simulink model "tb_adc_5g_spi_sys"  (Simulink 7.0)
settings: Solver=ode45  StartTime=0.0  StopTime=2000  RelTol=1e-3
libraries: xbsIndex_r4 x446, simulink x28, xps_library x12, dspsigops x12, xbsReplacements_r4 x4, casper_library x2
(part 2 of 5)

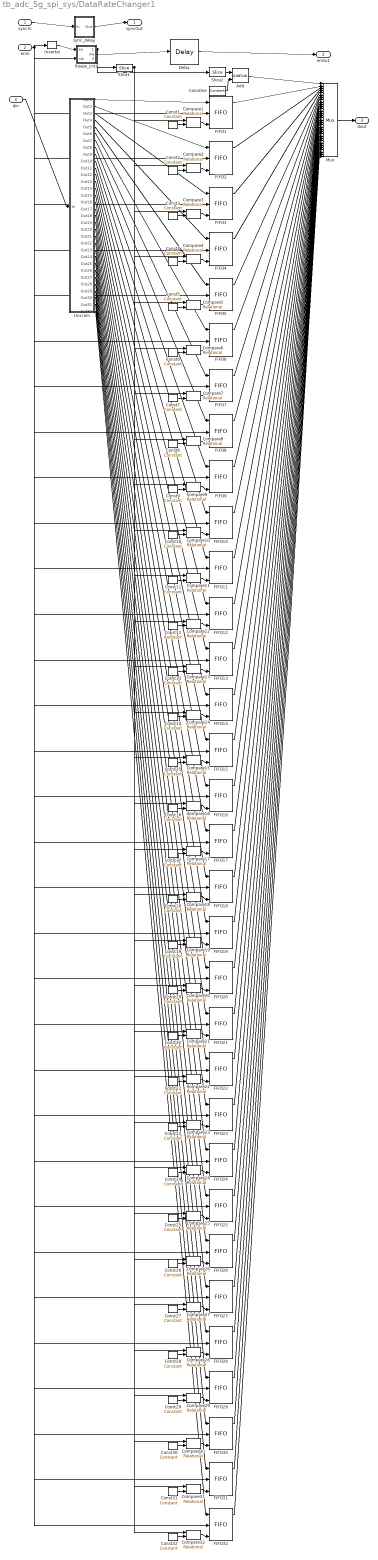
== system tb_adc_5g_spi_sys/DataRateChanger1 ==
  syncIn : Inport  OutDataType=sfix(16)  OutScaling=2^0
  enIn : Inport  Port=2  OutDataType=sfix(16)  OutScaling=2^0
  din : Inport  Port=3  OutDataType=sfix(16)  OutScaling=2^0
  Add : xbsIndex_r4/AddSub  mode=Addition  use_carryin=off  use_carryout=off  en=off  latency=0  precision=User Defined  arith_type=Unsigned  n_bits=5  bin_pt=0  quantization=Truncate  overflow=Wrap  dbl_ovrd=off  use_behavioral_HDL=off  pipelined=off  use_rpm=on  hw_selection=Fabric  block_type=addsub
      settings: block_version=10.1.3
  Compare{1..32} (32 alike) : xbsIndex_r4/Relational  mode=a=b  en=off  latency=0  dbl_ovrd=off  block_type=relational
      Compare1 settings: xl_area=[0, 0, 0, 0, 0, 0, 0]  block_version=10.1.2
      Compare10 settings: block_version=10.1.3
      Compare11 settings: block_version=10.1.3
      Compare12 settings: block_version=10.1.3
      Compare13 settings: block_version=10.1.3
      Compare14 settings: block_version=10.1.3
      Compare15 settings: block_version=10.1.3
      Compare16 settings: block_version=10.1.3
      Compare17 settings: block_version=10.1.3
      Compare18 settings: block_version=10.1.3
      Compare19 settings: block_version=10.1.3
      Compare2 settings: block_version=10.1.3
      Compare20 settings: block_version=10.1.3
      Compare21 settings: block_version=10.1.3
      Compare22 settings: block_version=10.1.3
      Compare23 settings: block_version=10.1.3
      Compare24 settings: block_version=10.1.3
      Compare25 settings: block_version=10.1.3
      Compare26 settings: block_version=10.1.3
      Compare27 settings: block_version=10.1.3
      Compare28 settings: block_version=10.1.3
      Compare29 settings: block_version=10.1.3
      Compare3 settings: block_version=10.1.3
      Compare30 settings: block_version=10.1.3
      Compare31 settings: block_version=10.1.3
      Compare32 settings: block_version=10.1.3
      Compare4 settings: block_version=10.1.3
      Compare5 settings: block_version=10.1.3
      Compare6 settings: block_version=10.1.3
      Compare7 settings: block_version=10.1.3
      Compare8 settings: block_version=10.1.3
      Compare9 settings: block_version=10.1.3
  ConsOne : xbsIndex_r4/Constant  arith_type=Unsigned  const=1  n_bits=1  bin_pt=0  explicit_period=off  period=1  equ=P=C  opselect=C  inp2=PCIN>>17  opr=+  inp1=P  carry=CIN  dbl_ovrd=off  block_type=constant
  Const1 : xbsIndex_r4/Constant  arith_type=Unsigned  const=1  n_bits=9  bin_pt=0  explicit_period=off  period=1  equ=P=C  opselect=C  inp2=PCIN>>17  opr=+  inp1=P  carry=CIN  dbl_ovrd=off  block_type=constant
      settings: block_version=10.1.2
  Const10 : xbsIndex_r4/Constant  arith_type=Unsigned  const=145  n_bits=9  bin_pt=0  explicit_period=off  period=1  equ=P=C  opselect=C  inp2=PCIN>>17  opr=+  inp1=P  carry=CIN  dbl_ovrd=off  block_type=constant
  Const11 : xbsIndex_r4/Constant  arith_type=Unsigned  const=161  n_bits=9  bin_pt=0  explicit_period=off  period=1  equ=P=C  opselect=C  inp2=PCIN>>17  opr=+  inp1=P  carry=CIN  dbl_ovrd=off  block_type=constant
  Const12 : xbsIndex_r4/Constant  arith_type=Unsigned  const=177  n_bits=9  bin_pt=0  explicit_period=off  period=1  equ=P=C  opselect=C  inp2=PCIN>>17  opr=+  inp1=P  carry=CIN  dbl_ovrd=off  block_type=constant
  Const13 : xbsIndex_r4/Constant  arith_type=Unsigned  const=193  n_bits=9  bin_pt=0  explicit_period=off  period=1  equ=P=C  opselect=C  inp2=PCIN>>17  opr=+  inp1=P  carry=CIN  dbl_ovrd=off  block_type=constant
  Const14 : xbsIndex_r4/Constant  arith_type=Unsigned  const=209  n_bits=9  bin_pt=0  explicit_period=off  period=1  equ=P=C  opselect=C  inp2=PCIN>>17  opr=+  inp1=P  carry=CIN  dbl_ovrd=off  block_type=constant
  Const15 : xbsIndex_r4/Constant  arith_type=Unsigned  const=225  n_bits=9  bin_pt=0  explicit_period=off  period=1  equ=P=C  opselect=C  inp2=PCIN>>17  opr=+  inp1=P  carry=CIN  dbl_ovrd=off  block_type=constant
  Const16 : xbsIndex_r4/Constant  arith_type=Unsigned  const=241  n_bits=9  bin_pt=0  explicit_period=off  period=1  equ=P=C  opselect=C  inp2=PCIN>>17  opr=+  inp1=P  carry=CIN  dbl_ovrd=off  block_type=constant
  Const17 : xbsIndex_r4/Constant  arith_type=Unsigned  const=257  n_bits=9  bin_pt=0  explicit_period=off  period=1  equ=P=C  opselect=C  inp2=PCIN>>17  opr=+  inp1=P  carry=CIN  dbl_ovrd=off  block_type=constant
  Const18 : xbsIndex_r4/Constant  arith_type=Unsigned  const=273  n_bits=9  bin_pt=0  explicit_period=off  period=1  equ=P=C  opselect=C  inp2=PCIN>>17  opr=+  inp1=P  carry=CIN  dbl_ovrd=off  block_type=constant
  Const19 : xbsIndex_r4/Constant  arith_type=Unsigned  const=289  n_bits=9  bin_pt=0  explicit_period=off  period=1  equ=P=C  opselect=C  inp2=PCIN>>17  opr=+  inp1=P  carry=CIN  dbl_ovrd=off  block_type=constant
  Const2 : xbsIndex_r4/Constant  arith_type=Unsigned  const=17  n_bits=9  bin_pt=0  explicit_period=off  period=1  equ=P=C  opselect=C  inp2=PCIN>>17  opr=+  inp1=P  carry=CIN  dbl_ovrd=off  block_type=constant
  Const20 : xbsIndex_r4/Constant  arith_type=Unsigned  const=305  n_bits=9  bin_pt=0  explicit_period=off  period=1  equ=P=C  opselect=C  inp2=PCIN>>17  opr=+  inp1=P  carry=CIN  dbl_ovrd=off  block_type=constant
  Const21 : xbsIndex_r4/Constant  arith_type=Unsigned  const=321  n_bits=9  bin_pt=0  explicit_period=off  period=1  equ=P=C  opselect=C  inp2=PCIN>>17  opr=+  inp1=P  carry=CIN  dbl_ovrd=off  block_type=constant
  Const22 : xbsIndex_r4/Constant  arith_type=Unsigned  const=337  n_bits=9  bin_pt=0  explicit_period=off  period=1  equ=P=C  opselect=C  inp2=PCIN>>17  opr=+  inp1=P  carry=CIN  dbl_ovrd=off  block_type=constant
  Const23 : xbsIndex_r4/Constant  arith_type=Unsigned  const=353  n_bits=9  bin_pt=0  explicit_period=off  period=1  equ=P=C  opselect=C  inp2=PCIN>>17  opr=+  inp1=P  carry=CIN  dbl_ovrd=off  block_type=constant
  Const24 : xbsIndex_r4/Constant  arith_type=Unsigned  const=369  n_bits=9  bin_pt=0  explicit_period=off  period=1  equ=P=C  opselect=C  inp2=PCIN>>17  opr=+  inp1=P  carry=CIN  dbl_ovrd=off  block_type=constant
  Const25 : xbsIndex_r4/Constant  arith_type=Unsigned  const=385  n_bits=9  bin_pt=0  explicit_period=off  period=1  equ=P=C  opselect=C  inp2=PCIN>>17  opr=+  inp1=P  carry=CIN  dbl_ovrd=off  block_type=constant
  Const26 : xbsIndex_r4/Constant  arith_type=Unsigned  const=401  n_bits=9  bin_pt=0  explicit_period=off  period=1  equ=P=C  opselect=C  inp2=PCIN>>17  opr=+  inp1=P  carry=CIN  dbl_ovrd=off  block_type=constant
  Const27 : xbsIndex_r4/Constant  arith_type=Unsigned  const=417  n_bits=9  bin_pt=0  explicit_period=off  period=1  equ=P=C  opselect=C  inp2=PCIN>>17  opr=+  inp1=P  carry=CIN  dbl_ovrd=off  block_type=constant
  Const28 : xbsIndex_r4/Constant  arith_type=Unsigned  const=433  n_bits=9  bin_pt=0  explicit_period=off  period=1  equ=P=C  opselect=C  inp2=PCIN>>17  opr=+  inp1=P  carry=CIN  dbl_ovrd=off  block_type=constant
  Const29 : xbsIndex_r4/Constant  arith_type=Unsigned  const=449  n_bits=9  bin_pt=0  explicit_period=off  period=1  equ=P=C  opselect=C  inp2=PCIN>>17  opr=+  inp1=P  carry=CIN  dbl_ovrd=off  block_type=constant
  Const3 : xbsIndex_r4/Constant  arith_type=Unsigned  const=33  n_bits=9  bin_pt=0  explicit_period=off  period=1  equ=P=C  opselect=C  inp2=PCIN>>17  opr=+  inp1=P  carry=CIN  dbl_ovrd=off  block_type=constant
  Const30 : xbsIndex_r4/Constant  arith_type=Unsigned  const=465  n_bits=9  bin_pt=0  explicit_period=off  period=1  equ=P=C  opselect=C  inp2=PCIN>>17  opr=+  inp1=P  carry=CIN  dbl_ovrd=off  block_type=constant
  Const31 : xbsIndex_r4/Constant  arith_type=Unsigned  const=481  n_bits=9  bin_pt=0  explicit_period=off  period=1  equ=P=C  opselect=C  inp2=PCIN>>17  opr=+  inp1=P  carry=CIN  dbl_ovrd=off  block_type=constant
  Const32 : xbsIndex_r4/Constant  arith_type=Unsigned  const=497  n_bits=9  bin_pt=0  explicit_period=off  period=1  equ=P=C  opselect=C  inp2=PCIN>>17  opr=+  inp1=P  carry=CIN  dbl_ovrd=off  block_type=constant
  Const4 : xbsIndex_r4/Constant  arith_type=Unsigned  const=49  n_bits=9  bin_pt=0  explicit_period=off  period=1  equ=P=C  opselect=C  inp2=PCIN>>17  opr=+  inp1=P  carry=CIN  dbl_ovrd=off  block_type=constant
  Const5 : xbsIndex_r4/Constant  arith_type=Unsigned  const=65  n_bits=9  bin_pt=0  explicit_period=off  period=1  equ=P=C  opselect=C  inp2=PCIN>>17  opr=+  inp1=P  carry=CIN  dbl_ovrd=off  block_type=constant
  Const6 : xbsIndex_r4/Constant  arith_type=Unsigned  const=81  n_bits=9  bin_pt=0  explicit_period=off  period=1  equ=P=C  opselect=C  inp2=PCIN>>17  opr=+  inp1=P  carry=CIN  dbl_ovrd=off  block_type=constant
  Const7 : xbsIndex_r4/Constant  arith_type=Unsigned  const=97  n_bits=9  bin_pt=0  explicit_period=off  period=1  equ=P=C  opselect=C  inp2=PCIN>>17  opr=+  inp1=P  carry=CIN  dbl_ovrd=off  block_type=constant
  Const8 : xbsIndex_r4/Constant  arith_type=Unsigned  const=113  n_bits=9  bin_pt=0  explicit_period=off  period=1  equ=P=C  opselect=C  inp2=PCIN>>17  opr=+  inp1=P  carry=CIN  dbl_ovrd=off  block_type=constant
  Const9 : xbsIndex_r4/Constant  arith_type=Unsigned  const=129  n_bits=9  bin_pt=0  explicit_period=off  period=1  equ=P=C  opselect=C  inp2=PCIN>>17  opr=+  inp1=P  carry=CIN  dbl_ovrd=off  block_type=constant
  Delay : xbsIndex_r4/Delay  en=off  latency=3  dbl_ovrd=off  reg_retiming=off  block_type=delay
      settings: block_version=10.1.2
  FIFO1 : xbsIndex_r4/FIFO  depth=16  percent_nbits=1  rst=off  en=off  use_dcount=off  use_almost_empty=off  almost_empty_thresh=2  use_almost_full=off  almost_full_thresh=14  dbl_ovrd=off  mem_type=Block RAM  explicit_period=off  period=1  block_type=fifo
      settings: xl_area=[0, 0, 0, 0, 0, 0, 0]  block_version=10.1.2
  FIFO{2..32} (31 alike) : xbsIndex_r4/FIFO  depth=16  percent_nbits=1  rst=off  en=off  use_dcount=off  use_almost_empty=off  almost_empty_thresh=2  use_almost_full=off  almost_full_thresh=14  dbl_ovrd=off  mem_type=Block RAM  block_type=fifo
      settings: block_version=10.1.3
  Inverter : xbsIndex_r4/Inverter  en=off  latency=0  dbl_ovrd=off  block_type=inv
      settings: xl_area=[0, 0, 0, 0, 0, 0, 0]  block_version=10.1.2
  Mux : xbsIndex_r4/Mux  inputs=32  en=off  latency=1  precision=Full  arith_type=Unsigned  n_bits=16  bin_pt=14  quantization=Truncate  overflow=Wrap  dbl_ovrd=off  block_type=mux
  Slice1 : xbsIndex_r4/Slice  nbits=9  boolean_output=off  mode=Lower Bit Location + Width  bit1=0  base1=MSB of Input  bit0=0  base0=LSB of Input  dbl_ovrd=off  block_type=slice
      settings: infoedit="Extracts a given range of bits from each input sample and presents it at the output.  The output type is ordinarily unsigned with binary point at zero, but can be Boolean when the slice is one bit wide.<P><P>Hardware notes: In hardware this block costs nothing."  block_version=10.1.2
  Slice2 : xbsIndex_r4/Slice  nbits=5  boolean_output=off  mode=Lower Bit Location + Width  bit1=0  base1=MSB of Input  bit0=4  base0=LSB of Input  dbl_ovrd=off  block_type=slice
      settings: infoedit="Extracts a given range of bits from each input sample and presents it at the output.  The output type is ordinarily unsigned with binary point at zero, but can be Boolean when the slice is one bit wide.<P><P>Hardware notes: In hardware this block costs nothing."  block_version=10.1.3
  Uncram : Subsystem  AncestorBlock=gavrt_library/uncram  mask(uncram){num_slice=32, slice_width=1, bin_pt=0, arith_type=0}
      mask prompts: num_slice "Number of slices"; slice_width "Slice Width"; bin_pt "Output Binary Point"; arith_type "Output Arithmetic Type (0=Unsigned, 1=Signed)"
      mask help: Takes a concatenated input and slices it up into even pieces and reinterprets them as signed fixed point numbers with a given binary point.
      mask init:
      | uncram_init(gcb, ...
      |     'num_slice', num_slice, ...
      |     'slice_width', slice_width, ...
      |     'bin_pt', bin_pt, ...
      |     'arith_type', arith_type);
      settings: AttributesFormatString=UFix_1_0
  freeze_cntr : Subsystem  AncestorBlock=casper_library/Misc/freeze_cntr  mask(freeze_cntr){CounterBits=10}
      mask prompts: CounterBits "Counter Length (2^?)"
      mask help:
      | A freeze counter is an enabled counter which holds its final value (regardless of enables)
      | until it is reset.
      mask Help: eval('xlWeb([getenv(''MLIB_ROOT''), ''\casper_library\doc\freeze_cntr_usage.html''])')
  sync_delay : Subsystem  AncestorBlock=casper_library/Delays/sync_delay  mask(sync_delay){DelayLen=5}
      mask prompts: DelayLen "Delay Length:"
      mask help: Delay an infrequent boolean pulse by the specified number of clocks.
      mask init:
      | BitWidth = max(2, ceil(log2(DelayLen+1)));
      | UseCounter = 1;
      | if DelayLen == 0,
      | 	UseCounter = 0;
      | end
      mask Help: eval('xlWeb([getenv(''MLIB_ROOT''), ''\casper_library\doc\sync_delay_usage.html''])')
      mask Display: fprintf('Z^-%d', DelayLen)
  syncOut : Outport  OutDataType=sfix(16)  OutScaling=2^0
  enOut : Outport  Port=2  OutDataType=sfix(16)  OutScaling=2^0
  dout : Outport  Port=3  OutDataType=sfix(16)  OutScaling=2^0
  wires:
  syncIn/1 -> sync_delay/1(In)
  sync_delay/1(Out) -> syncOut/1
  enIn/1 -> Inverter/1, freeze_cntr/2(rst), FIFO1/2, FIFO2/2, FIFO3/2, FIFO4/2, FIFO5/2, FIFO6/2, FIFO7/2, FIFO8/2, FIFO9/2, FIFO10/2, FIFO11/2, FIFO12/2, FIFO13/2, FIFO14/2, FIFO15/2, FIFO16/2, FIFO17/2, FIFO18/2, FIFO19/2, FIFO20/2, FIFO21/2, FIFO22/2, FIFO23/2, FIFO24/2, FIFO25/2, FIFO26/2, FIFO27/2, FIFO28/2, FIFO29/2, FIFO30/2, FIFO31/2, FIFO32/2
  Inverter/1 -> freeze_cntr/1(en)
  freeze_cntr/2(we) -> Delay/1
  Delay/1 -> enOut/1
  freeze_cntr/1(addr) -> Slice1/1, Slice2/1
  din/1 -> Uncram/1(In)
  Mux/1 -> dout/1
  Slice2/1 -> Add/1
  ConsOne/1 -> Add/2
  Add/1 -> Mux/1
  Const1/1 -> Compare1/2
  Compare1/1 -> FIFO1/3
  Uncram/1(Out1) -> FIFO1/1
  FIFO1/1 -> Mux/2
  Slice1/1 -> Compare1/1, Compare2/1, Compare3/1, Compare4/1, Compare5/1, Compare6/1, Compare7/1, Compare8/1, Compare9/1, Compare10/1, Compare11/1, Compare12/1, Compare13/1, Compare14/1, Compare15/1, Compare16/1, Compare17/1, Compare18/1, Compare19/1, Compare20/1, Compare21/1, Compare22/1, Compare23/1, Compare24/1, Compare25/1, Compare26/1, Compare27/1, Compare28/1, Compare29/1, Compare30/1, Compare31/1, Compare32/1
  Const2/1 -> Compare2/2
  Compare2/1 -> FIFO2/3
  Uncram/2(Out2) -> FIFO2/1
  FIFO2/1 -> Mux/3
  Const3/1 -> Compare3/2
  Compare3/1 -> FIFO3/3
  Uncram/3(Out3) -> FIFO3/1
  FIFO3/1 -> Mux/4
  Const4/1 -> Compare4/2
  Compare4/1 -> FIFO4/3
  Uncram/4(Out4) -> FIFO4/1
  FIFO4/1 -> Mux/5
  Const5/1 -> Compare5/2
  Compare5/1 -> FIFO5/3
  Uncram/5(Out5) -> FIFO5/1
  FIFO5/1 -> Mux/6
  Const6/1 -> Compare6/2
  Compare6/1 -> FIFO6/3
  Uncram/6(Out6) -> FIFO6/1
  FIFO6/1 -> Mux/7
  Const7/1 -> Compare7/2
  Compare7/1 -> FIFO7/3
  Uncram/7(Out7) -> FIFO7/1
  FIFO7/1 -> Mux/8
  Const8/1 -> Compare8/2
  Compare8/1 -> FIFO8/3
  Uncram/8(Out8) -> FIFO8/1
  FIFO8/1 -> Mux/9
  Const9/1 -> Compare9/2
  Compare9/1 -> FIFO9/3
  Uncram/9(Out9) -> FIFO9/1
  FIFO9/1 -> Mux/10
  Const10/1 -> Compare10/2
  Compare10/1 -> FIFO10/3
  Uncram/10(Out10) -> FIFO10/1
  FIFO10/1 -> Mux/11
  Const11/1 -> Compare11/2
  Compare11/1 -> FIFO11/3
  Uncram/11(Out11) -> FIFO11/1
  FIFO11/1 -> Mux/12
  Const12/1 -> Compare12/2
  Compare12/1 -> FIFO12/3
  Uncram/12(Out12) -> FIFO12/1
  FIFO12/1 -> Mux/13
  Const13/1 -> Compare13/2
  Compare13/1 -> FIFO13/3
  Uncram/13(Out13) -> FIFO13/1
  FIFO13/1 -> Mux/14
  Const14/1 -> Compare14/2
  Compare14/1 -> FIFO14/3
  Uncram/14(Out14) -> FIFO14/1
  FIFO14/1 -> Mux/15
  Const15/1 -> Compare15/2
  Compare15/1 -> FIFO15/3
  Uncram/15(Out15) -> FIFO15/1
  FIFO15/1 -> Mux/16
  Const16/1 -> Compare16/2
  Compare16/1 -> FIFO16/3
  Uncram/16(Out16) -> FIFO16/1
  FIFO16/1 -> Mux/17
  Const17/1 -> Compare17/2
  Compare17/1 -> FIFO17/3
  Uncram/17(Out17) -> FIFO17/1
  FIFO17/1 -> Mux/18
  Const18/1 -> Compare18/2
  Compare18/1 -> FIFO18/3
  Uncram/18(Out18) -> FIFO18/1
  FIFO18/1 -> Mux/19
  Const19/1 -> Compare19/2
  Compare19/1 -> FIFO19/3
  Uncram/19(Out19) -> FIFO19/1
  FIFO19/1 -> Mux/20
  Const20/1 -> Compare20/2
  Compare20/1 -> FIFO20/3
  Uncram/20(Out20) -> FIFO20/1
  FIFO20/1 -> Mux/21
  Const21/1 -> Compare21/2
  Compare21/1 -> FIFO21/3
  Uncram/21(Out21) -> FIFO21/1
  FIFO21/1 -> Mux/22
  Const22/1 -> Compare22/2
  Compare22/1 -> FIFO22/3
  Uncram/22(Out22) -> FIFO22/1
  FIFO22/1 -> Mux/23
  Const23/1 -> Compare23/2
  Compare23/1 -> FIFO23/3
  Uncram/23(Out23) -> FIFO23/1
  FIFO23/1 -> Mux/24
  Const24/1 -> Compare24/2
  Compare24/1 -> FIFO24/3
  Uncram/24(Out24) -> FIFO24/1
  FIFO24/1 -> Mux/25
  Const25/1 -> Compare25/2
  Compare25/1 -> FIFO25/3
  Uncram/25(Out25) -> FIFO25/1
  FIFO25/1 -> Mux/26
  Const26/1 -> Compare26/2
  Compare26/1 -> FIFO26/3
  Uncram/26(Out26) -> FIFO26/1
  FIFO26/1 -> Mux/27
  Const27/1 -> Compare27/2
  Compare27/1 -> FIFO27/3
  Uncram/27(Out27) -> FIFO27/1
  FIFO27/1 -> Mux/28
  Const28/1 -> Compare28/2
  Compare28/1 -> FIFO28/3
  Uncram/28(Out28) -> FIFO28/1
  FIFO28/1 -> Mux/29
  Const29/1 -> Compare29/2
  Compare29/1 -> FIFO29/3
  Uncram/29(Out29) -> FIFO29/1
  FIFO29/1 -> Mux/30
  Const30/1 -> Compare30/2
  Compare30/1 -> FIFO30/3
  Uncram/30(Out30) -> FIFO30/1
  FIFO30/1 -> Mux/31
  Const31/1 -> Compare31/2
  Compare31/1 -> FIFO31/3
  Uncram/31(Out31) -> FIFO31/1
  FIFO31/1 -> Mux/32
  Const32/1 -> Compare32/2
  Compare32/1 -> FIFO32/3
  Uncram/32(Out32) -> FIFO32/1
  FIFO32/1 -> Mux/33

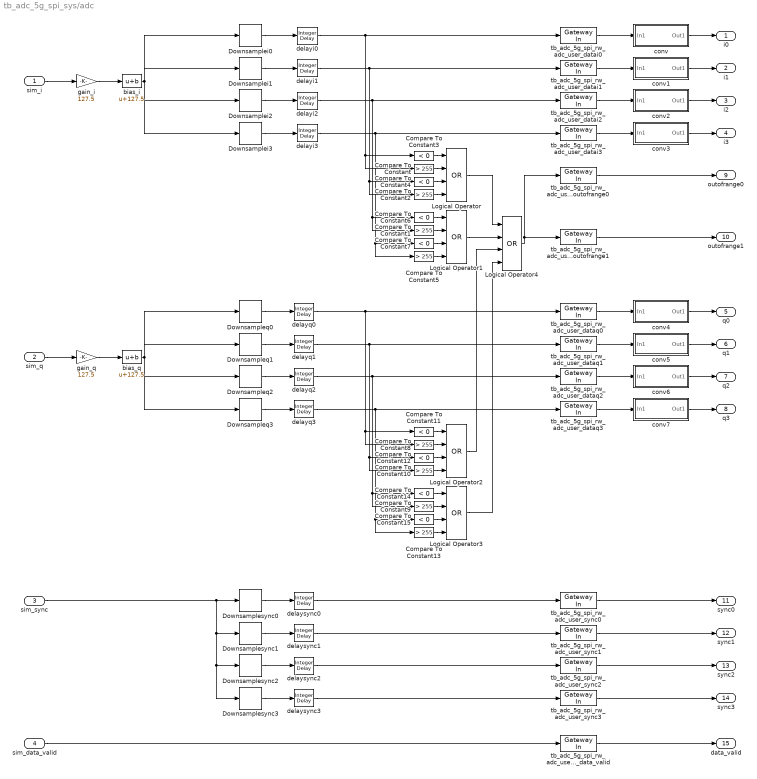
== system tb_adc_5g_spi_sys/adc ==
  sim_i : Inport  SampleTime=sample_period/4
  sim_q : Inport  Port=2  SampleTime=sample_period/4
  sim_sync : Inport  Port=3  SampleTime=sample_period/4  OutDataType=sfix(16)  OutScaling=2^0
  sim_data_valid : Inport  Port=4  SampleTime=sample_period/4  OutDataType=sfix(16)  OutScaling=2^0
  Compare To Constant{,1..2,5,8..10,13} (8 alike) : simulink/Logic and Bit Operations/Compare To Constant  SystemSampleTime=-1  relop=>  const=255  LogicOutDataTypeMode=boolean  ZeroCross=off
  Compare To Constant{3..4,6..7,11..12,14..15} (8 alike) : simulink/Logic and Bit Operations/Compare To Constant  SystemSampleTime=-1  relop=<  const=0  LogicOutDataTypeMode=boolean  ZeroCross=off
  Downsamplei0 : dspsigops/Downsample  N=4  phase=0  ic=0  smode=Allow multirate  fmode=Maintain input frame size
  Downsamplei1 : dspsigops/Downsample  N=4  phase=1  ic=0  smode=Allow multirate  fmode=Maintain input frame size
  Downsamplei2 : dspsigops/Downsample  N=4  phase=2  ic=0  smode=Allow multirate  fmode=Maintain input frame size
  Downsamplei3 : dspsigops/Downsample  N=4  phase=3  ic=0  smode=Allow multirate  fmode=Maintain input frame size
  Downsampleq0 : dspsigops/Downsample  N=4  phase=0  ic=0  smode=Allow multirate  fmode=Maintain input frame size
  Downsampleq1 : dspsigops/Downsample  N=4  phase=1  ic=0  smode=Allow multirate  fmode=Maintain input frame size
  Downsampleq2 : dspsigops/Downsample  N=4  phase=2  ic=0  smode=Allow multirate  fmode=Maintain input frame size
  Downsampleq3 : dspsigops/Downsample  N=4  phase=3  ic=0  smode=Allow multirate  fmode=Maintain input frame size
  Downsamplesync0 : dspsigops/Downsample  N=4  phase=0  ic=0  smode=Allow multirate  fmode=Maintain input frame size
  Downsamplesync1 : dspsigops/Downsample  N=4  phase=1  ic=0  smode=Allow multirate  fmode=Maintain input frame size
  Downsamplesync2 : dspsigops/Downsample  N=4  phase=2  ic=0  smode=Allow multirate  fmode=Maintain input frame size
  Downsamplesync3 : dspsigops/Downsample  N=4  phase=3  ic=0  smode=Allow multirate  fmode=Maintain input frame size
  Logical Operator{,1..4} (5 alike) : Logic  Operator=OR  Inputs=4  AllPortsSameDT=off  OutDataTypeMode=boolean
  bias_i : Bias  Bias=127.5  SaturateOnIntegerOverflow=on
  bias_q : Bias  Bias=127.5  SaturateOnIntegerOverflow=on
  conv : Subsystem
  conv1 : Subsystem
  conv2 : Subsystem
  conv3 : Subsystem
  conv4 : Subsystem
  conv5 : Subsystem
  conv6 : Subsystem
  conv7 : Subsystem
  delayi0 : simulink/Discrete/Integer Delay  vinit=0.0  samptime=-1  NumDelays=2
  delayi1 : simulink/Discrete/Integer Delay  vinit=0.0  samptime=-1  NumDelays=1
  delayi2 : simulink/Discrete/Integer Delay  vinit=0.0  samptime=-1  NumDelays=1
  delayi3 : simulink/Discrete/Integer Delay  vinit=0.0  samptime=-1  NumDelays=1
  delayq0 : simulink/Discrete/Integer Delay  vinit=0.0  samptime=-1  NumDelays=2
  delayq1 : simulink/Discrete/Integer Delay  vinit=0.0  samptime=-1  NumDelays=1
  delayq2 : simulink/Discrete/Integer Delay  vinit=0.0  samptime=-1  NumDelays=1
  delayq3 : simulink/Discrete/Integer Delay  vinit=0.0  samptime=-1  NumDelays=1
  delaysync0 : simulink/Discrete/Integer Delay  vinit=0.0  samptime=-1  NumDelays=2
  delaysync1 : simulink/Discrete/Integer Delay  vinit=0.0  samptime=-1  NumDelays=1
  delaysync2 : simulink/Discrete/Integer Delay  vinit=0.0  samptime=-1  NumDelays=1
  delaysync3 : simulink/Discrete/Integer Delay  vinit=0.0  samptime=-1  NumDelays=1
  gain_i : Gain  Gain=127.5  SaturateOnIntegerOverflow=on
  gain_q : Gain  Gain=127.5  SaturateOnIntegerOverflow=on
  tb_adc_5g_spi_rw_adc_user_data_valid : xbsIndex_r4/Gateway In  arith_type=Boolean  n_bits=8  bin_pt=0  quantization="Round  (unbiased: +/- Inf)"  overflow=Saturate  period=sample_period  dbl_ovrd=off  timing_constraint=None  locs_specified=off  LOCs={}  block_type=gatewayin
      settings: infoedit="Gateway in block.  Converts inputs of type Simulink integer, double and fixed point to  Xilinx fixed point type.<P><P>Hardware notes:  In hardware these blocks become top level input ports."  xl_area=[0 0 0 0 8 0 0]  block_version=8.2.02
  tb_adc_5g_spi_rw_adc_user_datai{0..3} (4 alike) : xbsIndex_r4/Gateway In  arith_type=Unsigned  n_bits=8  bin_pt=0  quantization="Round  (unbiased: +/- Inf)"  overflow=Saturate  period=sample_period  dbl_ovrd=off  timing_constraint=None  locs_specified=off  LOCs={}  block_type=gatewayin
      settings: infoedit="Gateway in block.  Converts inputs of type Simulink integer, double and fixed point to  Xilinx fixed point type.<P><P>Hardware notes:  In hardware these blocks become top level input ports."  xl_area=[0 0 0 0 8 0 0]  block_version=8.2.02
  tb_adc_5g_spi_rw_adc_user_dataq{0..3} (4 alike) : xbsIndex_r4/Gateway In  arith_type=Unsigned  n_bits=8  bin_pt=0  quantization="Round  (unbiased: +/- Inf)"  overflow=Saturate  period=sample_period  dbl_ovrd=off  timing_constraint=None  locs_specified=off  LOCs={}  block_type=gatewayin
      settings: infoedit="Gateway in block.  Converts inputs of type Simulink integer, double and fixed point to  Xilinx fixed point type.<P><P>Hardware notes:  In hardware these blocks become top level input ports."  xl_area=[0 0 0 0 8 0 0]  block_version=8.2.02
  tb_adc_5g_spi_rw_adc_user_outofrange0 : xbsIndex_r4/Gateway In  arith_type=Boolean  n_bits=8  bin_pt=0  quantization="Round  (unbiased: +/- Inf)"  overflow=Saturate  period=sample_period  dbl_ovrd=off  timing_constraint=None  locs_specified=off  LOCs={}  block_type=gatewayin
      settings: infoedit="Gateway in block.  Converts inputs of type Simulink integer, double and fixed point to  Xilinx fixed point type.<P><P>Hardware notes:  In hardware these blocks become top level input ports."  xl_area=[0 0 0 0 8 0 0]  block_version=8.2.02
  tb_adc_5g_spi_rw_adc_user_outofrange1 : xbsIndex_r4/Gateway In  arith_type=Boolean  n_bits=8  bin_pt=0  quantization="Round  (unbiased: +/- Inf)"  overflow=Saturate  period=sample_period  dbl_ovrd=off  timing_constraint=None  locs_specified=off  LOCs={}  block_type=gatewayin
      settings: infoedit="Gateway in block.  Converts inputs of type Simulink integer, double and fixed point to  Xilinx fixed point type.<P><P>Hardware notes:  In hardware these blocks become top level input ports."  xl_area=[0 0 0 0 8 0 0]  block_version=8.2.02
  tb_adc_5g_spi_rw_adc_user_sync{0..3} (4 alike) : xbsIndex_r4/Gateway In  arith_type=Boolean  n_bits=8  bin_pt=0  quantization="Round  (unbiased: +/- Inf)"  overflow=Saturate  period=sample_period  dbl_ovrd=off  timing_constraint=None  locs_specified=off  LOCs={}  block_type=gatewayin
      settings: infoedit="Gateway in block.  Converts inputs of type Simulink integer, double and fixed point to  Xilinx fixed point type.<P><P>Hardware notes:  In hardware these blocks become top level input ports."  xl_area=[0 0 0 0 8 0 0]  block_version=8.2.02
  i0 : Outport  OutDataType=sfix(16)  OutScaling=2^0
  i1 : Outport  Port=2  OutDataType=sfix(16)  OutScaling=2^0
  i2 : Outport  Port=3  OutDataType=sfix(16)  OutScaling=2^0
  i3 : Outport  Port=4  OutDataType=sfix(16)  OutScaling=2^0
  q0 : Outport  Port=5  OutDataType=sfix(16)  OutScaling=2^0
  q1 : Outport  Port=6  OutDataType=sfix(16)  OutScaling=2^0
  q2 : Outport  Port=7  OutDataType=sfix(16)  OutScaling=2^0
  q3 : Outport  Port=8  OutDataType=sfix(16)  OutScaling=2^0
  outofrange0 : Outport  Port=9  OutDataType=sfix(16)  OutScaling=2^0
  outofrange1 : Outport  Port=10  OutDataType=sfix(16)  OutScaling=2^0
  sync0 : Outport  Port=11  OutDataType=sfix(16)  OutScaling=2^0
  sync1 : Outport  Port=12  OutDataType=sfix(16)  OutScaling=2^0
  sync2 : Outport  Port=13  OutDataType=sfix(16)  OutScaling=2^0
  sync3 : Outport  Port=14  OutDataType=sfix(16)  OutScaling=2^0
  data_valid : Outport  Port=15  OutDataType=sfix(16)  OutScaling=2^0
  wires:
  tb_adc_5g_spi_rw_adc_user_datai0/1 -> conv/1(In1)
  sim_data_valid/1 -> tb_adc_5g_spi_rw_adc_user_data_valid/1
  tb_adc_5g_spi_rw_adc_user_data_valid/1 -> data_valid/1
  tb_adc_5g_spi_rw_adc_user_sync3/1 -> sync3/1
  tb_adc_5g_spi_rw_adc_user_sync2/1 -> sync2/1
  delaysync3/1 -> tb_adc_5g_spi_rw_adc_user_sync3/1
  delaysync2/1 -> tb_adc_5g_spi_rw_adc_user_sync2/1
  Downsamplesync3/1 -> delaysync3/1
  Downsamplesync2/1 -> delaysync2/1
  tb_adc_5g_spi_rw_adc_user_sync1/1 -> sync1/1
  delaysync0/1 -> tb_adc_5g_spi_rw_adc_user_sync0/1
  Downsamplesync1/1 -> delaysync1/1
  Downsamplesync0/1 -> delaysync0/1
  sim_sync/1 -> Downsamplesync3/1, Downsamplesync2/1, Downsamplesync1/1, Downsamplesync0/1
  Compare To Constant5/1 -> Logical Operator1/4
  Compare To Constant7/1 -> Logical Operator1/3
  Compare To Constant1/1 -> Logical Operator1/2
  Compare To Constant6/1 -> Logical Operator1/1
  Compare To Constant2/1 -> Logical Operator/4
  Compare To Constant4/1 -> Logical Operator/3
  Compare To Constant/1 -> Logical Operator/2
  Compare To Constant3/1 -> Logical Operator/1
  tb_adc_5g_spi_rw_adc_user_outofrange1/1 -> outofrange1/1
  delayq0/1 -> tb_adc_5g_spi_rw_adc_user_dataq0/1, Compare To Constant8/1, Compare To Constant11/1
  Downsampleq0/1 -> delayq0/1
  delayi0/1 -> Compare To Constant3/1, Compare To Constant/1, tb_adc_5g_spi_rw_adc_user_datai0/1
  Downsamplei1/1 -> delayi1/1
  Downsamplei2/1 -> delayi2/1
  Downsamplei3/1 -> delayi3/1
  Downsampleq1/1 -> delayq1/1
  Downsampleq2/1 -> delayq2/1
  Downsampleq3/1 -> delayq3/1
  tb_adc_5g_spi_rw_adc_user_datai1/1 -> conv1/1(In1)
  tb_adc_5g_spi_rw_adc_user_datai2/1 -> conv2/1(In1)
  tb_adc_5g_spi_rw_adc_user_datai3/1 -> conv3/1(In1)
  tb_adc_5g_spi_rw_adc_user_outofrange0/1 -> outofrange0/1
  tb_adc_5g_spi_rw_adc_user_sync0/1 -> sync0/1
  conv/1(Out1) -> i0/1
  conv1/1(Out1) -> i1/1
  conv2/1(Out1) -> i2/1
  conv3/1(Out1) -> i3/1
  tb_adc_5g_spi_rw_adc_user_dataq0/1 -> conv4/1(In1)
  conv4/1(Out1) -> q0/1
  tb_adc_5g_spi_rw_adc_user_dataq1/1 -> conv5/1(In1)
  conv5/1(Out1) -> q1/1
  tb_adc_5g_spi_rw_adc_user_dataq2/1 -> conv6/1(In1)
  conv6/1(Out1) -> q2/1
  tb_adc_5g_spi_rw_adc_user_dataq3/1 -> conv7/1(In1)
  conv7/1(Out1) -> q3/1
  Downsamplei0/1 -> delayi0/1
  delayi1/1 -> Compare To Constant4/1, Compare To Constant2/1, tb_adc_5g_spi_rw_adc_user_datai1/1
  delayi2/1 -> Compare To Constant1/1, Compare To Constant6/1, tb_adc_5g_spi_rw_adc_user_datai2/1
  delayi3/1 -> Compare To Constant5/1, Compare To Constant7/1, tb_adc_5g_spi_rw_adc_user_datai3/1
  delayq1/1 -> Compare To Constant10/1, Compare To Constant12/1, tb_adc_5g_spi_rw_adc_user_dataq1/1
  delayq2/1 -> Compare To Constant9/1, Compare To Constant14/1, tb_adc_5g_spi_rw_adc_user_dataq2/1
  delayq3/1 -> Compare To Constant13/1, Compare To Constant15/1, tb_adc_5g_spi_rw_adc_user_dataq3/1
  delaysync1/1 -> tb_adc_5g_spi_rw_adc_user_sync1/1
  Compare To Constant11/1 -> Logical Operator2/1
  Compare To Constant13/1 -> Logical Operator3/4
  Compare To Constant15/1 -> Logical Operator3/3
  Compare To Constant9/1 -> Logical Operator3/2
  Compare To Constant14/1 -> Logical Operator3/1
  Compare To Constant10/1 -> Logical Operator2/4
  Compare To Constant12/1 -> Logical Operator2/3
  Compare To Constant8/1 -> Logical Operator2/2
  Logical Operator4/1 -> tb_adc_5g_spi_rw_adc_user_outofrange0/1, tb_adc_5g_spi_rw_adc_user_outofrange1/1
  Logical Operator/1 -> Logical Operator4/1
  Logical Operator1/1 -> Logical Operator4/2
  Logical Operator2/1 -> Logical Operator4/3
  Logical Operator3/1 -> Logical Operator4/4
  sim_i/1 -> gain_i/1
  gain_i/1 -> bias_i/1
  bias_i/1 -> Downsamplei0/1, Downsamplei1/1, Downsamplei2/1, Downsamplei3/1
  sim_q/1 -> gain_q/1
  gain_q/1 -> bias_q/1
  bias_q/1 -> Downsampleq0/1, Downsampleq1/1, Downsampleq2/1, Downsampleq3/1
